simulink model "Six_DoF_Dynamics_Test"  (R2020a)
settings: Solver=VariableStepAuto  StartTime=0.0  StopTime=P.t_end  RelTol=1e-3
InitFcn:
  | drone_param
StartFcn:
  | drone_param
undefined symbols (not defined in the file or in its folder): drawDrone, P
libraries: simulink x4
ContinueFcn:
  | FT2frfl
settings Model: Creator=sadam  LastModifiedBy=Adam
settings DataIOCC: ReturnWorkspaceOutputs=off
settings DebuggingCC: ArithmeticOperatorsInVariantConditions=warning
settings SFSimCC: SimUseLocalCustomCode=off  CustomCodeUndefinedFunction=UseInterfaceOnly
settings RTWCC: RTWUseLocalCustomCode=off

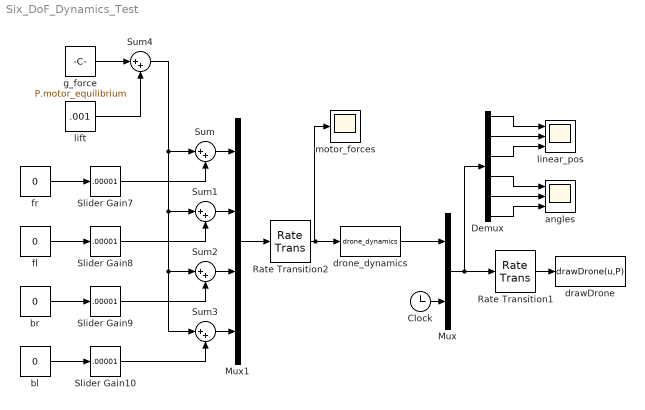
== system Six_DoF_Dynamics_Test ==
  Clock : Clock
  Demux : Demux  Outputs=6
  Mux : Mux  Inputs=2
  Mux1 : Mux
  Rate Transition1 : RateTransition  OutPortSampleTime=P.t_plot
  Rate Transition2 : RateTransition  OutPortSampleTime=P.Ts
  Slider Gain{7..10} (4 alike) : simulink/Math Operations/Slider Gain  gain=.00001  low=-5  high=10
  Sum{,1..4} (5 alike) : Sum  Inputs=|++
  angles : Scope  NumInputPorts=3
  bl : Constant  Value=0
  br : Constant  Value=0
  drawDrone : MATLABFcn  MATLABFcn=drawDrone(u,P)  OutputDimensions=0
  drone_dynamics : S-Function  FunctionName=drone_dynamics  Parameters=P  SFunctionDeploymentMode=off  EnableBusSupport=off
  fl : Constant  Value=0
  fr : Constant  Value=0
  g_force : Constant  Value=P.motor_equilibrium
  lift : Constant  Value=.001
  linear_pos : Scope  NumInputPorts=3
  motor_forces : Scope
  wires:
  Rate Transition1/1 -> drawDrone/1
  drone_dynamics/1 -> Mux/1
  fr/1 -> Slider Gain7/1
  bl/1 -> Slider Gain10/1
  br/1 -> Slider Gain9/1
  fl/1 -> Slider Gain8/1
  Clock/1 -> Mux/2
  Mux/1 -> Demux/1, Rate Transition1/1
  Sum/1 -> Mux1/1
  Sum3/1 -> Mux1/4
  Sum2/1 -> Mux1/3
  Sum1/1 -> Mux1/2
  Slider Gain7/1 -> Sum/2
  Slider Gain8/1 -> Sum1/2
  Slider Gain9/1 -> Sum2/2
  Slider Gain10/1 -> Sum3/2
  Rate Transition2/1 -> motor_forces/1, drone_dynamics/1
  Mux1/1 -> Rate Transition2/1
  g_force/1 -> Sum4/1
  Sum4/1 -> Sum1/1, Sum3/1, Sum2/1, Sum/1
  lift/1 -> Sum4/2
  Demux/1 -> linear_pos/1
  Demux/2 -> linear_pos/2
  Demux/3 -> linear_pos/3
  Demux/4 -> angles/1
  Demux/5 -> angles/2
  Demux/6 -> angles/3
